simulink model "Zdc_VSI_v_loop"  (Simulink 8.2)
settings: Solver=ode23t  StartTime=0.0  StopTime=0.5  MaxStep=25e-6  RelTol=1e-4  AbsTol=1e-5
values from neighbouring files (symbols this model uses):
  C = 1*31.5e-6    (= 3.15e-05)    [TVSI_vil_tf_cal_sim_comp_frd_model.m]    (also in VSI_ol_init.m = 3.13e-05; VSI_ol_tf_cal_sim_comp_frd_model.m = 3.13e-05; Zac_VSI.m = 3.18e-05; Zdc_VSI.m)
  Gdel = Gsvm    [TVSI_vil_tf_cal_sim_comp_frd_model.m]    (also in VSI_ol_init.m; VSI_ol_tf_cal_sim_comp_frd_model.m; Zac_VSI.m; Zdc_VSI.m)
  Ki = tf_filter_dq    [TVSI_vil_tf_cal_sim_comp_frd_model.m]    (also in VSI_ol_init.m; Zac_VSI.m; Zdc_VSI.m)
  kii = Kii_VSI/270    (= 0)    [TVSI_vil_tf_cal_sim_comp_frd_model.m]    (also in Zac_VSI.m; Zdc_VSI.m = 121.0095)
  kiv = Kiv_VSI    (= 523.598775598)    [TVSI_vil_tf_cal_sim_comp_frd_model.m]    (also in Zac_VSI.m = 78.5398163397; Zdc_VSI.m = 130.8997)
  kpi = Kpi_VSI/270    (= 0.0116355283466)    [TVSI_vil_tf_cal_sim_comp_frd_model.m]    (also in Zac_VSI.m = 0.00407243492132; Zdc_VSI.m = 0.0465)
  kpv = Kpv_VSI    (= 0.197920337176)    [TVSI_vil_tf_cal_sim_comp_frd_model.m]    (also in Zac_VSI.m = 0.0290283161192; Zdc_VSI.m = 0.0495)
  Kv = tf_filter_dq    [TVSI_vil_tf_cal_sim_comp_frd_model.m]    (also in VSI_ol_init.m; Zac_VSI.m; Zdc_VSI.m)
  L = 1.0e-3    (= 0.001)    [TVSI_vil_tf_cal_sim_comp_frd_model.m]    (also in VSI_ol_init.m; VSI_ol_tf_cal_sim_comp_frd_model.m; Zac_VSI.m = 0.000506643235509; Zdc_VSI.m)
  R = 12    [TVSI_vil_tf_cal_sim_comp_frd_model.m]    (also in VSI_ol_init.m = 15; VSI_ol_tf_cal_sim_comp_frd_model.m = 12000; Zac_VSI.m; Zdc_VSI.m)
  RL = 0.13    [TVSI_vil_tf_cal_sim_comp_frd_model.m]    (also in VSI_ol_init.m = 0.15; VSI_ol_tf_cal_sim_comp_frd_model.m = 0.15; Zac_VSI.m = 0.06; Zdc_VSI.m)
  Vdc = 270    [TVSI_vil_tf_cal_sim_comp_frd_model.m]    (also in VSI_ol_init.m; VSI_ol_tf_cal_sim_comp_frd_model.m; Zac_VSI.m; Zdc_VSI.m)
  Vdref = Vsdq(1)    [TVSI_vil_tf_cal_sim_comp_frd_model.m]    (also in VSI_ol_init.m; VSI_ol_tf_cal_sim_comp_frd_model.m; Zac_VSI.m; Zdc_VSI.m)
  Vqref = Vsdq(2)    [TVSI_vil_tf_cal_sim_comp_frd_model.m]    (also in VSI_ol_init.m; VSI_ol_tf_cal_sim_comp_frd_model.m; Zac_VSI.m; Zdc_VSI.m)
  w = 500*2*pi    (= 3141.59265359)    [JF_CMOD.m]    (also in JF_SMOD.m; TVSI_vil_tf_cal_sim_comp_frd_model.m = 376.991118431; VSI_ol_init.m = 2513.27412287; VSI_ol_tf_cal_sim_comp_frd_model.m = 376.991118431)
libraries: powerlib x24, cstblocks x12
settings Model: Creator=marko  LastModifiedBy=wenbo  BufferReuse=off
settings OptimizationCC: BlockReduction=off  InlineParams=on  BufferReuse=off
settings DebuggingCC: AlgebraicLoopMsg=none  SolverPrmCheckMsg=none  UnconnectedInputMsg=none  UnconnectedOutputMsg=none  UnconnectedLineMsg=none

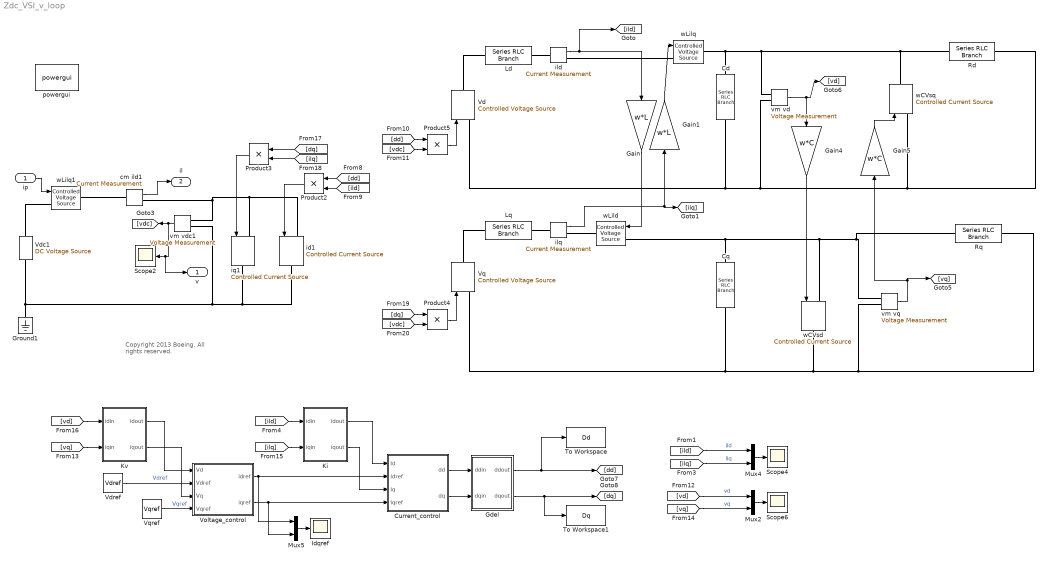
== system Zdc_VSI_v_loop ==
  note: Copyright 2013 Boeing. All rights reserved.
  ip : Inport
  Cd : powerlib/Elements/Series RLC Branch  LConnTagsString=__new0  RConnTagsString=__new0  BranchType=C  Resistance=1  Inductance=1e-3  SetiL0=off  InitialCurrent=0  Capacitance=C  Setx0=off  InitialVoltage=0  Measurements=None
  Cq : powerlib/Elements/Series RLC Branch  LConnTagsString=__new0  RConnTagsString=__new0  BranchType=C  Resistance=1  Inductance=1e-3  SetiL0=off  InitialCurrent=0  Capacitance=C  Setx0=off  InitialVoltage=0  Measurements=None
  Current_control : Subsystem
  Gain : Gain  Gain=w*L
  Gain1 : Gain  Gain=w*L
  Gain4 : Gain  Gain=w*C
  Gain5 : Gain  Gain=w*C
  Gdel : Subsystem
  Ground1 : powerlib/Elements/Ground  LConnTagsString=a
  Idqref : Scope
      settings: YMin=4.4  YMax=5.35  SaveName=ildq_matlab8
  Ki : Subsystem
  Kv : Subsystem
  Ld : powerlib/Elements/Series RLC Branch  LConnTagsString=__new0  RConnTagsString=__new0  BranchType=RL  Resistance=RL  Inductance=L  SetiL0=off  InitialCurrent=0  Capacitance=1e-6  Setx0=off  InitialVoltage=0  Measurements=None
  Lq : powerlib/Elements/Series RLC Branch  LConnTagsString=__new0  RConnTagsString=__new0  BranchType=RL  Resistance=RL  Inductance=L  SetiL0=off  InitialCurrent=0  Capacitance=1e-6  Setx0=off  InitialVoltage=0  Measurements=None
  Mux2 : Mux  Inputs=2
  Mux4 : Mux  Inputs=2
  Mux5 : Mux  Inputs=2
  Product{2..5} (4 alike) : Product  RndMeth=Zero
  Rd : powerlib/Elements/Series RLC Branch  LConnTagsString=__new0  RConnTagsString=__new0  BranchType=R  Resistance=R  Inductance=1e-3  SetiL0=off  InitialCurrent=0  Capacitance=1e-6  Setx0=off  InitialVoltage=0  Measurements=None
  Rq : powerlib/Elements/Series RLC Branch  LConnTagsString=__new0  RConnTagsString=__new0  BranchType=R  Resistance=R  Inductance=1e-3  SetiL0=off  InitialCurrent=0  Capacitance=1e-6  Setx0=off  InitialVoltage=0  Measurements=None
  Scope2 : Scope
      settings: YMin=270  YMax=270  SaveName=ildq_matlab1
  Scope4 : Scope
      settings: YMin=-0.25  YMax=5.25  SaveName=ildq_matlab3
  Scope6 : Scope
      settings: YMin=-10  YMax=130  SaveName=ildq_matlab4
  To Workspace : ToWorkspace  VariableName=Dd  SampleTime=-1
  To Workspace1 : ToWorkspace  VariableName=Dq  SampleTime=-1
  Vd : powerlib/Electrical Sources/Controlled Voltage Source  Initialize=on  Source_Type=DC  Amplitude=0  Phase=0  Frequency=0  Measurements=None
  Vdc1 : powerlib/Electrical Sources/DC Voltage Source  Amplitude=Vdc  Measurements=None
  Vdref : Constant  Value=Vdref
  Voltage_control : Subsystem
  Vq : powerlib/Electrical Sources/Controlled Voltage Source  Initialize=on  Source_Type=DC  Amplitude=0  Phase=0  Frequency=0  Measurements=None
  Vqref : Constant  Value=Vqref
  cm ild1 : powerlib/Measurements/Current Measurement  PhasorSimulation=off  OutputType=Complex  PSBequivalent=0
  id1 : powerlib/Electrical Sources/Controlled Current Source  Initialize=on  Source_Type=DC  Amplitude=0  Phase=0  Frequency=0  Measurements=None
  ild : powerlib/Measurements/Current Measurement  PhasorSimulation=off  OutputType=Complex  PSBequivalent=0
  ilq : powerlib/Measurements/Current Measurement  PhasorSimulation=off  OutputType=Complex  PSBequivalent=0
  iq1 : powerlib/Electrical Sources/Controlled Current Source  Initialize=on  Source_Type=DC  Amplitude=0  Phase=0  Frequency=0  Measurements=None
  powergui : powerlib/powergui  Priority=1  SimulationMode=Continuous  SolverType=Tustin  SampleTime=50e-6  frequency=60  SPID=off  DisableSnubberDevices=off  DisableRonSwitches=off  DisableVfSwitches=off  SwTol=0  Interpol=off  DisplayEquations=off  frequencyindice=0  Pbase=100e6  ErrMax=1e-4  Iterations=50  UnitsV=kV  UnitsW=MW  FunctionMessages=off  echomessages=off  HookPort=off  EnableUseOfTLC=off  x0status=blocks  RestoreLinks=warning  ResistiveCurrentMeasurement=off  Frange=[0:2:500]  Ylog=off  Xlog=on  ShowGrid=off  save=off  variable=ZData  ZoomFFT=on  StartTime=0.0  cycles=1  DisplayStyle=1  fundamental=60  FreqAxis=off  MaxFrequency=1000  frequencyindicesteady=1  RmsSteady=1  display=off  Ts=0  methode=off
  vm vd : powerlib/Measurements/Voltage Measurement  PhasorSimulation=off  OutputType=Complex  PSBequivalent=0
  vm vdc1 : powerlib/Measurements/Voltage Measurement  PhasorSimulation=off  OutputType=Complex  PSBequivalent=0
  vm vq : powerlib/Measurements/Voltage Measurement  PhasorSimulation=off  OutputType=Complex  PSBequivalent=0
  wCVsd : powerlib/Electrical Sources/Controlled Current Source  Initialize=on  Source_Type=DC  Amplitude=0  Phase=0  Frequency=0  Measurements=None
  wCVsq : powerlib/Electrical Sources/Controlled Current Source  Initialize=on  Source_Type=DC  Amplitude=0  Phase=0  Frequency=0  Measurements=None
  wLild : powerlib/Electrical Sources/Controlled Voltage Source  Initialize=on  Source_Type=DC  Amplitude=0  Phase=0  Frequency=0  Measurements=None
  wLilq : powerlib/Electrical Sources/Controlled Voltage Source  Initialize=on  Source_Type=DC  Amplitude=0  Phase=0  Frequency=0  Measurements=None
  wLilq1 : powerlib/Electrical Sources/Controlled Voltage Source  Initialize=on  Source_Type=DC  Amplitude=0  Phase=0  Frequency=0  Measurements=None
  v : Outport
  il : Outport  Port=2
  wires:
  [ild] -> Mux4/1  "ild"
  [ilq] -> Mux4/2  "ilq"
  Mux4/1 -> Scope4/1
  [vd] -> Mux2/1  "vd"
  [vq] -> Mux2/2  "vq"
  Mux2/1 -> Scope6/1
  Voltage_control/2(iqref) -> Mux5/2, Current_control/4(Iqref)
  Gdel/1(ddout) -> [dd], To Workspace/1
  Gdel/2(dqout) -> [dq], To Workspace1/1
  Vqref/1 -> Voltage_control/4(Vqref)  "Vqref"
  Vdref/1 -> Voltage_control/2(Vdref)  "Vdref"
  Voltage_control/1(idref) -> Mux5/1, Current_control/2(Idref)
  Mux5/1 -> Idqref/1
  [ild] -> Ki/1(idin)
  [ilq] -> Ki/2(iqin)
  Ki/1(idout) -> Current_control/1(Id)
  Ki/2(iqout) -> Current_control/3(Iq)
  Current_control/1(dd) -> Gdel/1(ddin)
  Current_control/2(dq) -> Gdel/2(dqin)
  [vd] -> Kv/1(idin)
  [vq] -> Kv/2(iqin)
  Kv/1(idout) -> Voltage_control/1(Vd)
  Kv/2(iqout) -> Voltage_control/3(Vq)
  Product3/1 -> iq1/1
  [dq] -> Product4/1
  [vdc] -> Product4/2
  Product4/1 -> Vq/1
  [dd] -> Product5/1
  [vdc] -> Product5/2
  Product5/1 -> Vd/1
  vm vd/1 -> [vd], Gain4/1
  vm vq/1 -> Gain5/1, [vq]
  vm vdc1/1 -> [vdc], v/1, Scope2/1
  ilq/1 -> [ilq], Gain1/1
  ild/1 -> Gain/1, [ild]
  Gain5/1 -> wCVsq/1
  [dd] -> Product2/1
  [ild] -> Product2/2
  [dq] -> Product3/1
  [ilq] -> Product3/2
  Product2/1 -> id1/1
  Gain/1 -> wLild/1
  Gain1/1 -> wLilq/1
  Gain4/1 -> wCVsd/1
  ip/1 -> wLilq1/1
  cm ild1/1 -> il/1
  connections:
  Vq/LConn1 -- Cq/RConn1 -- wCVsd/RConn1 -- Rq/RConn1 -- vm vq/LConn2
  iq1/RConn1 -- id1/RConn1 -- Vdc1/LConn1 -- Ground1/LConn1 -- vm vdc1/LConn2
  wLild/LConn1 -- Cq/LConn1 -- wCVsd/LConn1 -- Rq/LConn1 -- vm vq/LConn1
  id1/LConn1 -- iq1/LConn1 -- cm ild1/RConn1 -- vm vdc1/LConn1
  Cd/LConn1 -- wLilq/RConn1 -- wCVsq/RConn1 -- Rd/LConn1 -- vm vd/LConn1
  Vd/LConn1 -- Cd/RConn1 -- Rd/RConn1 -- wCVsq/LConn1 -- vm vd/LConn2
  wLild/RConn1 -- ilq/RConn1
  Lq/RConn1 -- Vq/RConn1
  Ld/LConn1 -- Vd/RConn1
  ild/LConn1 -- Ld/RConn1
  ilq/LConn1 -- Lq/LConn1
  wLilq/LConn1 -- ild/RConn1
  wLilq1/LConn1 -- Vdc1/RConn1
  cm ild1/LConn1 -- wLilq1/RConn1

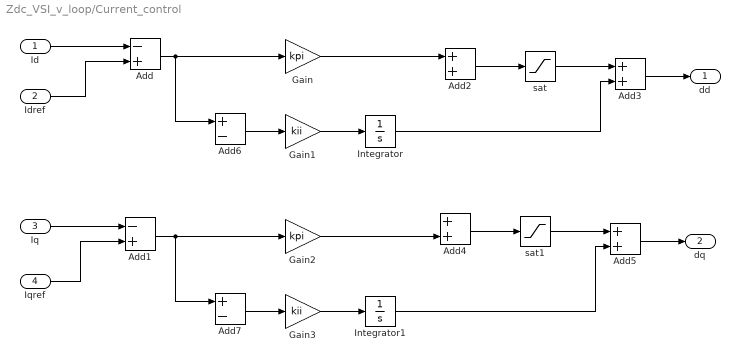
== system Zdc_VSI_v_loop/Current_control ==
  Id : Inport
  Idref : Inport  Port=2
  Iq : Inport  Port=3
  Iqref : Inport  Port=4
  Add : Sum  Inputs=-+
  Add1 : Sum  Inputs=-+
  Add{2..5} (4 alike) : Sum
  Add6 : Sum  Inputs=+-
  Add7 : Sum  Inputs=+-
  Gain : Gain  Gain=kpi
  Gain1 : Gain  Gain=kii
  Gain2 : Gain  Gain=kpi
  Gain3 : Gain  Gain=kii
  Integrator : Integrator
  Integrator1 : Integrator
  sat : Saturate  UpperLimit=1  LowerLimit=-1
  sat1 : Saturate  UpperLimit=1  LowerLimit=-1
  dd : Outport
  dq : Outport  Port=2
  wires:
  Id/1 -> Add/1
  Idref/1 -> Add/2
  Iq/1 -> Add1/1
  Iqref/1 -> Add1/2
  Add/1 -> Gain/1, Add6/1
  Gain1/1 -> Integrator/1
  Add2/1 -> sat/1
  sat/1 -> Add3/1
  Integrator/1 -> Add3/2
  Gain/1 -> Add2/1
  Add1/1 -> Gain2/1, Add7/1
  Gain3/1 -> Integrator1/1
  Gain2/1 -> Add4/2
  Add4/1 -> sat1/1
  sat1/1 -> Add5/1
  Integrator1/1 -> Add5/2
  Add5/1 -> dq/1
  Add6/1 -> Gain1/1
  Add7/1 -> Gain3/1
  Add3/1 -> dd/1

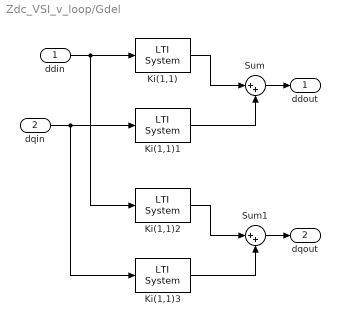
== system Zdc_VSI_v_loop/Gdel ==
  ddin : Inport
  dqin : Inport  Port=2
  Ki(1,1) : cstblocks/LTI System  sys=Gdel(1,1)  IC=[]
  Ki(1,1)1 : cstblocks/LTI System  sys=Gdel(1,2)  IC=[]
  Ki(1,1)2 : cstblocks/LTI System  sys=Gdel(2,1)  IC=[]
  Ki(1,1)3 : cstblocks/LTI System  sys=Gdel(2,2)  IC=[]
  Sum : Sum  Inputs=|++
  Sum1 : Sum  Inputs=|++
  ddout : Outport
  dqout : Outport  Port=2
  wires:
  Ki(1,1)/1 -> Sum/1
  Ki(1,1)1/1 -> Sum/2
  Ki(1,1)2/1 -> Sum1/1
  Ki(1,1)3/1 -> Sum1/2
  ddin/1 -> Ki(1,1)/1, Ki(1,1)2/1
  dqin/1 -> Ki(1,1)1/1, Ki(1,1)3/1
  Sum/1 -> ddout/1
  Sum1/1 -> dqout/1

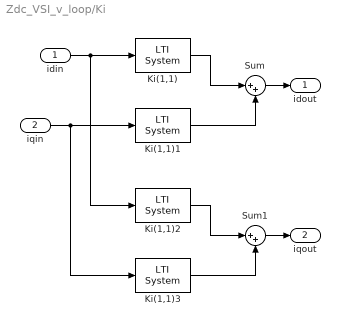
== system Zdc_VSI_v_loop/Ki ==
  idin : Inport
  iqin : Inport  Port=2
  Ki(1,1) : cstblocks/LTI System  sys=Ki(1,1)  IC=[]
  Ki(1,1)1 : cstblocks/LTI System  sys=Ki(1,2)  IC=[]
  Ki(1,1)2 : cstblocks/LTI System  sys=Ki(2,1)  IC=[]
  Ki(1,1)3 : cstblocks/LTI System  sys=Ki(2,2)  IC=[]
  Sum : Sum  Inputs=|++
  Sum1 : Sum  Inputs=|++
  idout : Outport
  iqout : Outport  Port=2
  wires:
  Ki(1,1)/1 -> Sum/1
  Ki(1,1)1/1 -> Sum/2
  Ki(1,1)2/1 -> Sum1/1
  Ki(1,1)3/1 -> Sum1/2
  idin/1 -> Ki(1,1)/1, Ki(1,1)2/1
  iqin/1 -> Ki(1,1)1/1, Ki(1,1)3/1
  Sum/1 -> idout/1
  Sum1/1 -> iqout/1

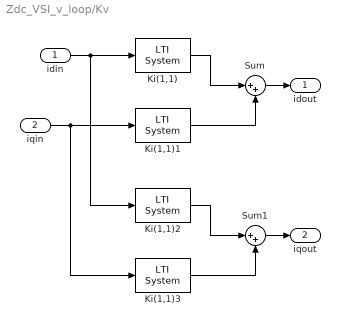
== system Zdc_VSI_v_loop/Kv ==
  idin : Inport
  iqin : Inport  Port=2
  Ki(1,1) : cstblocks/LTI System  sys=Kv(1,1)  IC=[]
  Ki(1,1)1 : cstblocks/LTI System  sys=Kv(1,2)  IC=[]
  Ki(1,1)2 : cstblocks/LTI System  sys=Kv(2,1)  IC=[]
  Ki(1,1)3 : cstblocks/LTI System  sys=Kv(2,2)  IC=[]
  Sum : Sum  Inputs=|++
  Sum1 : Sum  Inputs=|++
  idout : Outport
  iqout : Outport  Port=2
  wires:
  Sum1/1 -> iqout/1
  Sum/1 -> idout/1
  iqin/1 -> Ki(1,1)3/1, Ki(1,1)1/1
  idin/1 -> Ki(1,1)2/1, Ki(1,1)/1
  Ki(1,1)3/1 -> Sum1/2
  Ki(1,1)2/1 -> Sum1/1
  Ki(1,1)1/1 -> Sum/2
  Ki(1,1)/1 -> Sum/1

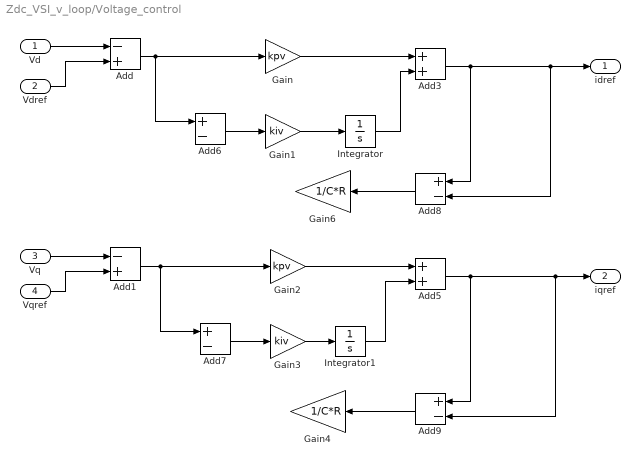
== system Zdc_VSI_v_loop/Voltage_control ==
  Vd : Inport
  Vdref : Inport  Port=2
  Vq : Inport  Port=3
  Vqref : Inport  Port=4
  Add : Sum  Inputs=-+
  Add1 : Sum  Inputs=-+
  Add3 : Sum
  Add5 : Sum
  Add{6..9} (4 alike) : Sum  Inputs=+-
  Gain : Gain  Gain=kpv
  Gain1 : Gain  Gain=kiv
  Gain2 : Gain  Gain=kpv
  Gain3 : Gain  Gain=kiv
  Gain4 : Gain  Gain=1/C*R
  Gain6 : Gain  Gain=1/C*R
  Integrator : Integrator
  Integrator1 : Integrator
  idref : Outport
  iqref : Outport  Port=2
  wires:
  Add9/1 -> Gain4/1
  Add8/1 -> Gain6/1
  Add3/1 -> Add8/1, idref/1, Add8/2
  Add7/1 -> Gain3/1
  Add6/1 -> Gain1/1
  Add5/1 -> Add9/1, iqref/1, Add9/2
  Integrator1/1 -> Add5/2
  Gain2/1 -> Add5/1
  Gain3/1 -> Integrator1/1
  Add1/1 -> Add7/1, Gain2/1
  Gain/1 -> Add3/1
  Integrator/1 -> Add3/2
  Gain1/1 -> Integrator/1
  Add/1 -> Add6/1, Gain/1
  Vqref/1 -> Add1/2
  Vq/1 -> Add1/1
  Vdref/1 -> Add/2
  Vd/1 -> Add/1
